simulink model "Siseslab2"  (R2022b)
settings: Solver=VariableStepAuto  StartTime=0.0  StopTime=10  MaxStep=.0001  RelTol=1e-3
values from neighbouring files (symbols this model uses):
  g = 9.81    [Practica_1.m]
  i1 = 0.3    [Practica_1.m]
  i2 = 0.25    [Practica_1.m]
  m1 = 0.2    [Practica_1.m]
  m2 = 0.1    [Practica_1.m]
settings Model: Creator=mluser  LastModifiedBy=mluser

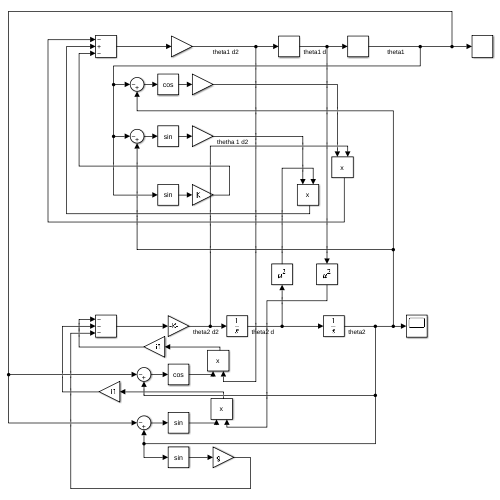
[thumbnail: Simulink's stored preview of the top-level diagram]
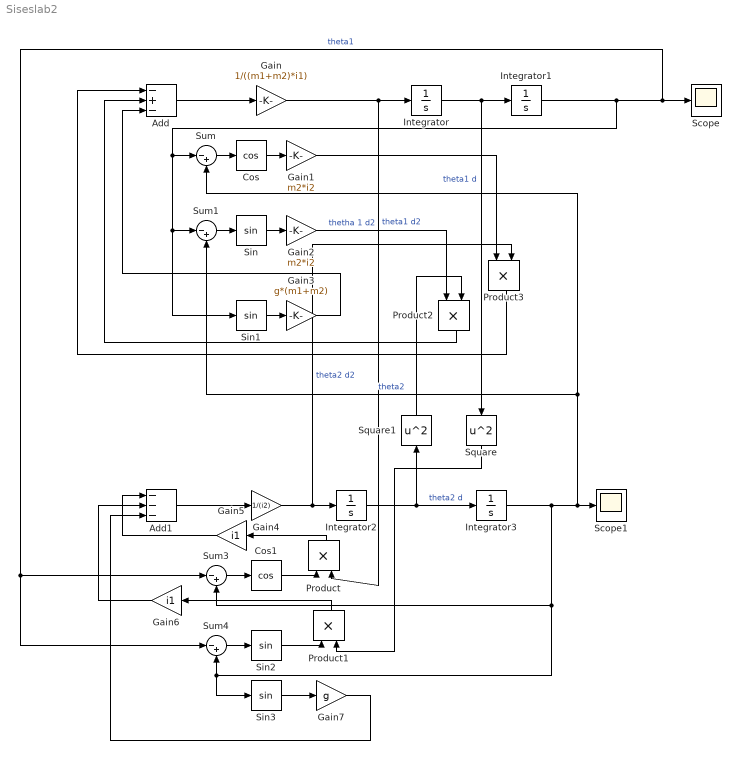
== system Siseslab2 ==
  Add : Sum  Inputs=-+-
  Add1 : Sum  Inputs=---
  Cos : Trigonometry  Operator=cos
  Cos1 : Trigonometry  Operator=cos
  Gain : Gain  Gain=1/((m1+m2)*i1)
  Gain1 : Gain  Gain=m2*i2
  Gain2 : Gain  Gain=m2*i2
  Gain3 : Gain  Gain=g*(m1+m2)
  Gain4 : Gain  Gain=1/(i2)
  Gain5 : Gain  Gain=i1
  Gain6 : Gain  Gain=i1
  Gain7 : Gain  Gain=g
  Integrator : Integrator
  Integrator1 : Integrator
  Integrator2 : Integrator
  Integrator3 : Integrator  InitialCondition=(35*pi)/180
  Product{,1..3} (4 alike) : Product
  Scope : Scope
  Scope1 : Scope
  Sin{,1..3} (4 alike) : Trigonometry
  Square : Math  Operator=square
  Square1 : Math  Operator=square
  Sum{,1,3..4} (4 alike) : Sum  Inputs=|-+
  wires:
  Integrator/1 -> Square/1, Integrator1/1  "theta1 d"
  Gain/1 -> Integrator/1, Product/2  "theta1 d2"
  Add/1 -> Gain/1
  Gain1/1 -> Product3/1
  Gain3/1 -> Add/3
  Sin1/1 -> Gain3/1
  Sin/1 -> Gain2/1
  Cos/1 -> Gain1/1
  Sum/1 -> Cos/1
  Sum1/1 -> Sin/1
  Integrator1/1 -> Sin1/1, Sum1/1, Sum/1, Sum4/1, Sum3/1, Scope/1  "theta1"
  Gain2/1 -> Product2/1  "thetha 1 d2"
  Integrator2/1 -> Square1/1, Integrator3/1  "theta2 d"
  Gain4/1 -> Integrator2/1, Product3/2  "theta2 d2"
  Add1/1 -> Gain4/1
  Sum3/1 -> Cos1/1
  Sum4/1 -> Sin2/1
  Integrator3/1 -> Sum/2, Sum1/2, Scope1/1, Sum3/2, Sum4/2, Sin3/1  "theta2"
  Cos1/1 -> Product/1
  Sin2/1 -> Product1/1
  Sin3/1 -> Gain7/1
  Gain7/1 -> Add1/3
  Product/1 -> Gain5/1
  Product1/1 -> Gain6/1
  Product2/1 -> Add/2
  Product3/1 -> Add/1
  Square/1 -> Product1/2
  Square1/1 -> Product2/2
  Gain5/1 -> Add1/1
  Gain6/1 -> Add1/2
